simulink model "SpaceFlexibleRobotLoadAug"  (R2025b)
settings: Solver=VariableStepAuto  StartTime=0.0  StopTime=10.0  RelTol=1e-3
undefined symbols (not defined in the file): DAP0, Ignew, InvDyn, InvDynAug, Jr, ra_norm, sig4, uls, ureal, uss, uw, XI
libraries: RCTblocks x210, SDTlibV2 x5
(part 1 of 4)
settings Model: Creator=T.FORMOSA  LastModifiedBy=andre
settings SolverCC: AlgebraicLoopSolver=TrustRegion
settings DebuggingCC: AlgebraicLoopMsg=none  UnconnectedInputMsg=warning  UnconnectedOutputMsg=warning  UnconnectedLineMsg=warning  ArithmeticOperatorsInVariantConditions=warning
settings ModelReferenceCC: EnableRefExpFcnMdlSchedulingChecks=on
settings SFSimCC: CustomCodeUndefinedFunction=UseInterfaceOnly
settings RTWCC: GPUComputeCapability=3.5  DLArmComputeVersion=19.05

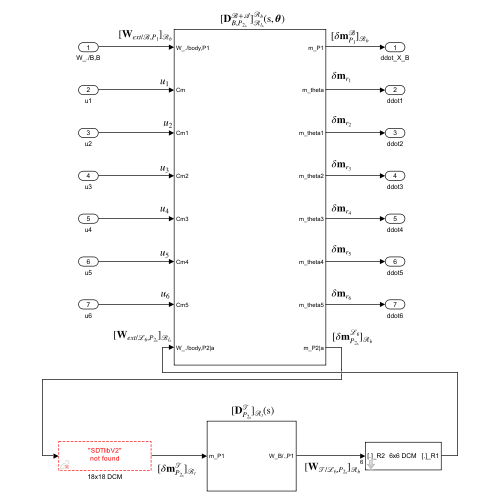
[thumbnail: Simulink's stored preview of the top-level diagram]
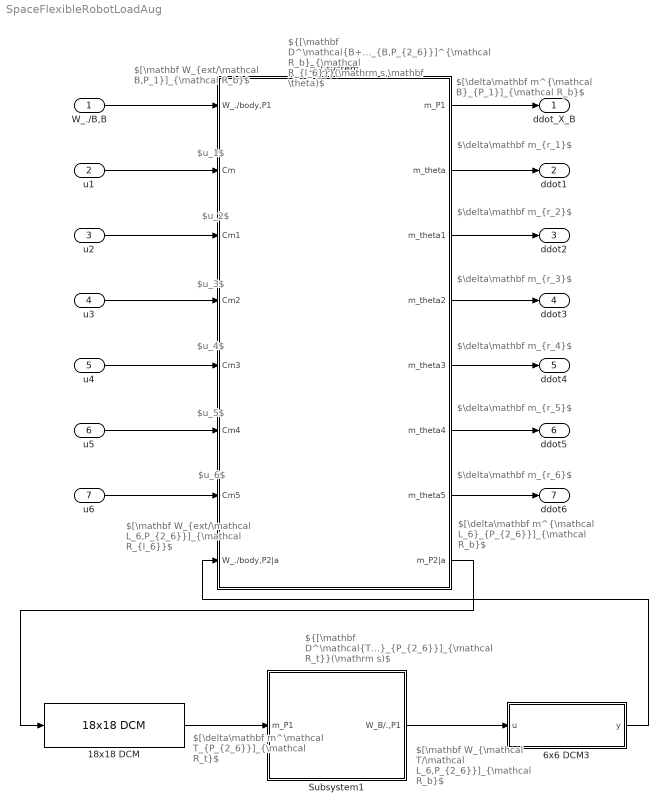
== system SpaceFlexibleRobotLoadAug ==
  note: $[\mathbf W_{ext/\mathcal B,P_1}]_{\mathcal R_b}$
  note: $[\delta\mathbf m^{\mathcal B}_{P_1}]_{\mathcal R_b}$
  note: $u_1$
  note: $\delta\mathbf m_{r_1}$
  note: $u_2$
  note: $u_3$
  note: $u_4$
  note: $u_5$
  note: $u_6$
  note: $[\mathbf W_{ext/\mathcal L_6,P_{2_6}}]_{\mathcal R_{l_6}}$
  note: $\delta\mathbf m_{r_2}$
  note: $\delta\mathbf m_{r_3}$
  note: $\delta\mathbf m_{r_4}$
  note: $\delta\mathbf m_{r_5}$
  note: $\delta\mathbf m_{r_6}$
  note: $[\delta\mathbf m^{\mathcal L_6}_{P_{2_6}}]_{\mathcal R_b}$
  note: ${[\mathbf D^\mathcal{B+A}_{B,P_{2_6}}]^{\mathcal R_b}_{\mathcal R_{l_6}}}(\mathrm s,\mathbf \theta)$
  note: $[\mathbf W_{\mathcal T/\mathcal L_6,P_{2_6}}]_{\mathcal R_b}$
  note: $[\delta\mathbf m^\mathcal T_{P_{2_6}}]_{\mathcal R_t}$
  note: ${[\mathbf D^\mathcal{T}_{P_{2_6}}]_{\mathcal R_t}}(\mathrm s)$
  W_./B,B : Inport
  u1 : Inport  Port=2
  u2 : Inport  Port=3
  u3 : Inport  Port=4
  u4 : Inport  Port=5
  u5 : Inport  Port=6
  u6 : Inport  Port=7
  18x18 DCM : SDTlibV2/3//6//18 DCM/18x18 DCM  rot=[0 0 1;-1 0 0;0 -1 0]  transp=on
      settings: SourceProductName=SDTlib
  6x6 DCM3 : Subsystem  mask(6x6 Direction cosine matrix (DCM)){rot=[0 0 1;-1 0 0;0 -1 0], transp=off}
      mask prompts: rot "3x3 DCM"; transp "Matrix transposed"
      mask help:
      | For 6 d.o.f. body motion (3 translations and 3 rotations), this block Implement the 6x6 rotation matrix (or its transposed) for a given 3x3 DCM.
      |
      | Considering 2 frames R1 and  R2, the DCM between R1 and R2 is defined as the 3x3 matrix where each column is the component vector of each R2 orthogonal unit vector expressed in R1. Thus
      |
      |    [v]_R1 = DCM  * [v]_R2.
      mask init:
      | if transp,
      |     rot=rot';
      | end
      mask Help: web('Doc6dcm.html','-browser')
      mask Display:
      | disp('6x6 DCM')
      | if transp
      |     port_label('input', 1, '[.]_R1')
      |     port_label('output', 1, '[.]_R2')
      | else
      |     port_label('input', 1, '[.]_R2')
      |     port_label('output', 1, '[.]_R1')
      | end
  Subsystem : Subsystem
  Subsystem1 : Subsystem
  ddot_X_B : Outport  VectorParamsAs1DForOutWhenUnconnected=off
  ddot1 : Outport  Port=2  VectorParamsAs1DForOutWhenUnconnected=off
  ddot2 : Outport  Port=3  VectorParamsAs1DForOutWhenUnconnected=off
  ddot3 : Outport  Port=4  VectorParamsAs1DForOutWhenUnconnected=off
  ddot4 : Outport  Port=5  VectorParamsAs1DForOutWhenUnconnected=off
  ddot5 : Outport  Port=6  VectorParamsAs1DForOutWhenUnconnected=off
  ddot6 : Outport  Port=7  VectorParamsAs1DForOutWhenUnconnected=off
  wires:
  W_./B,B/1 -> Subsystem/1(W_./body,P1)
  u1/1 -> Subsystem/2(Cm)
  u2/1 -> Subsystem/3(Cm1)
  u3/1 -> Subsystem/4(Cm2)
  u4/1 -> Subsystem/5(Cm3)
  u5/1 -> Subsystem/6(Cm4)
  u6/1 -> Subsystem/7(Cm5)
  6x6 DCM3/1(y) -> Subsystem/8(W_./body,P2|a)
  Subsystem/1(m_P1) -> ddot_X_B/1
  Subsystem/2(m_theta) -> ddot1/1
  Subsystem/3(m_theta1) -> ddot2/1
  Subsystem/4(m_theta2) -> ddot3/1
  Subsystem/5(m_theta3) -> ddot4/1
  Subsystem/6(m_theta4) -> ddot5/1
  Subsystem/7(m_theta5) -> ddot6/1
  Subsystem/8(m_P2|a) -> 18x18 DCM/1
  Subsystem1/1(W_B/.,P1) -> 6x6 DCM3/1(u)
  18x18 DCM/1 -> Subsystem1/1(m_P1)

== system SpaceFlexibleRobotLoadAug/6x6 DCM3 ==
  u : Inport  PortDimensions=6
  Demux : Demux  Outputs=[3 3]
  Mux : Mux  Inputs=[3 3]
  rotation : Gain  Gain=rot  Multiplication=Matrix(K*u) (u vector)
  translation : Gain  Gain=rot  Multiplication=Matrix(K*u) (u vector)
  y : Outport  VectorParamsAs1DForOutWhenUnconnected=off
  wires:
  rotation/1 -> Mux/2
  translation/1 -> Mux/1
  Demux/1 -> translation/1
  u/1 -> Demux/1
  Mux/1 -> y/1
  Demux/2 -> rotation/1

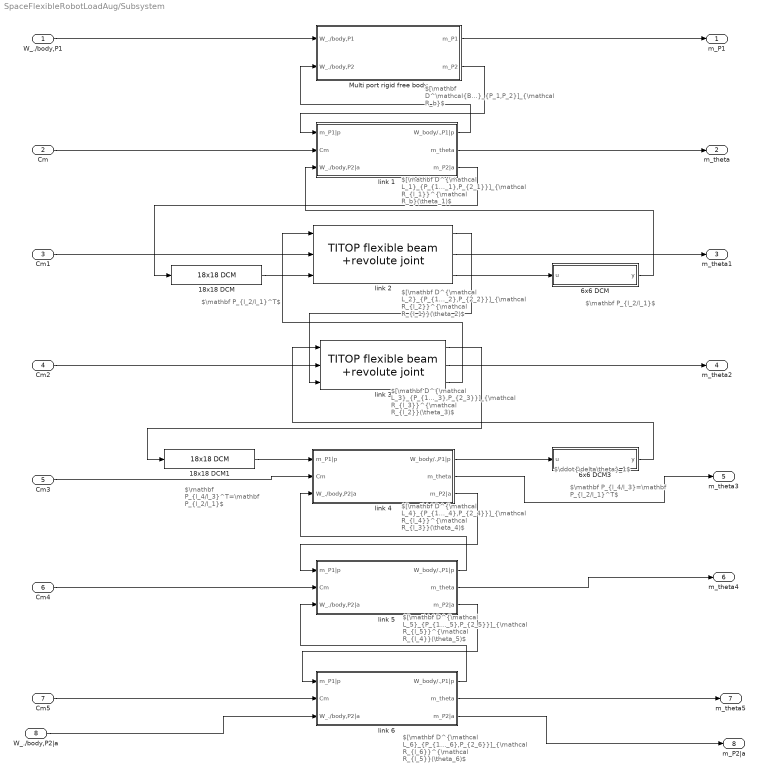
== system SpaceFlexibleRobotLoadAug/Subsystem ==
  note: $[\mathbf D^{\mathcal L_1}_{P_{1_1},P_{2_1}}]_{\mathcal R_{l_1}}^{\mathcal R_b}(\theta_1)$
  note: $[\mathbf D^\mathcal{B}_{P_1,P_2}]_{\mathcal R_b}$
  note: $\ddot{\delta\theta}_1$
  note: $[\mathbf D^{\mathcal L_2}_{P_{1_2},P_{2_2}}]_{\mathcal R_{l_2}}^{\mathcal R_{l_1}}(\theta_2)$
  note: $[\mathbf D^{\mathcal L_3}_{P_{1_3},P_{2_3}}]_{\mathcal R_{l_3}}^{\mathcal R_{l_2}}(\theta_3)$
  note: $[\mathbf D^{\mathcal L_4}_{P_{1_4},P_{2_4}}]_{\mathcal R_{l_4}}^{\mathcal R_{l_3}}(\theta_4)$
  note: $[\mathbf D^{\mathcal L_5}_{P_{1_5},P_{2_5}}]_{\mathcal R_{l_5}}^{\mathcal R_{l_4}}(\theta_5)$
  note: $[\mathbf D^{\mathcal L_6}_{P_{1_6},P_{2_6}}]_{\mathcal R_{l_6}}^{\mathcal R_{l_5}}(\theta_6)$
  note: $\mathbf P_{l_2/l_1}$
  note: $\mathbf P_{l_2/l_1}^T$
  note: $\mathbf P_{l_4/l_3}=\mathbf P_{l_2/l_1}^T$
  note: $\mathbf P_{l_4/l_3}^T=\mathbf P_{l_2/l_1}$
  W_./body,P1 : Inport
  Cm : Inport  Port=2
  Cm1 : Inport  Port=3
  Cm2 : Inport  Port=4
  Cm3 : Inport  Port=5
  Cm4 : Inport  Port=6
  Cm5 : Inport  Port=7
  W_./body,P2|a : Inport  Port=8
  18x18 DCM : SDTlibV2/3//6//18 DCM/18x18 DCM  rot=[0 1 0;-1 0 0;0 0 1]  transp=on
      settings: SourceProductName=SDTlib
  18x18 DCM1 : SDTlibV2/3//6//18 DCM/18x18 DCM  rot=[0 1 0;-1 0 0;0 0 1]  transp=off
      settings: SourceProductName=SDTlib
  6x6 DCM : Subsystem  mask(6x6 Direction cosine matrix (DCM)){rot=[0 1 0;-1 0 0;0 0 1], transp=off}
      mask prompts: rot "3x3 DCM"; transp "Matrix transposed"
      mask help:
      | For 6 d.o.f. body motion (3 translations and 3 rotations), this block Implement the 6x6 rotation matrix (or its transposed) for a given 3x3 DCM.
      |
      | Considering 2 frames R1 and  R2, the DCM between R1 and R2 is defined as the 3x3 matrix where each column is the component vector of each R2 orthogonal unit vector expressed in R1. Thus
      |
      |    [v]_R1 = DCM  * [v]_R2.
      mask init:
      | if transp,
      |     rot=rot';
      | end
      mask Help: web('Doc6dcm.html','-browser')
      mask Display:
      | disp('6x6 DCM')
      | if transp
      |     port_label('input', 1, '[.]_R1')
      |     port_label('output', 1, '[.]_R2')
      | else
      |     port_label('input', 1, '[.]_R2')
      |     port_label('output', 1, '[.]_R1')
      | end
  6x6 DCM3 : Subsystem  mask(6x6 Direction cosine matrix (DCM)){rot=[0 1 0;-1 0 0;0 0 1], transp=on}
      mask prompts: rot "3x3 DCM"; transp "Matrix transposed"
      mask help:
      | For 6 d.o.f. body motion (3 translations and 3 rotations), this block Implement the 6x6 rotation matrix (or its transposed) for a given 3x3 DCM.
      |
      | Considering 2 frames R1 and  R2, the DCM between R1 and R2 is defined as the 3x3 matrix where each column is the component vector of each R2 orthogonal unit vector expressed in R1. Thus
      |
      |    [v]_R1 = DCM  * [v]_R2.
      mask init:
      | if transp,
      |     rot=rot';
      | end
      mask Help: web('Doc6dcm.html','-browser')
      mask Display:
      | disp('6x6 DCM')
      | if transp
      |     port_label('input', 1, '[.]_R1')
      |     port_label('output', 1, '[.]_R2')
      | else
      |     port_label('input', 1, '[.]_R2')
      |     port_label('output', 1, '[.]_R1')
      | end
  Multi port rigid free body : Subsystem  mask(Multi-port rigid body (18nx6n)){m=1000, Ig=[666.6667 0 0; 0 666.6667 0; 0 0 666.6667], OG=[0;0;0], n=2, OP1=[0;0;0], OP2=[0;0;1], OP3=[ureal('P3_y',1,'percent',10);0;0], OP4=[0;0;0], OP5=[0;0;0]}
      mask prompts: m "Mass (Kg)"; Ig "Inertia (at G, Kg m^2)"; OG "OG (3x1 vector, m)"; n "Number of ports"; OP1 "OP1 (3x1 vector, m)"; OP2 "OP2 (3x1 vector, m)"; OP3 "OP3 (3x1 vector, m)"; OP4 "OP4 (3x1 vector, m)"; OP5 "OP5 (3x1 vector,m)"
      mask help:
      | 18nx6n dynamic model of a rigid body at n given points (ports) between wrenches applied at the n points (input) and the motions vectors at these points (output).
      |
      | 0: the reference point
      | G: the center of mass
      | Pi (i=1:n): the n given connection points (n<6).
      |
      | All parameters are expressed in the body frame.
      | Each parameter can be an uncertain parameter declared with "ureal"
      mask init:
      | MultiPortRigidFreeBody
      mask Help: web('Docmultiportrigidbase.html','-browser')
      mask TypeOptions n: 1 | 2 | 3 | 4 | 5
      mask DialogControl ParameterGroupVar Prompt: Main parameters
      mask DialogControl port1 Prompt: Port #1
      mask DialogControl port2 Prompt: #2
      mask DialogControl port3 Prompt: #3
      mask DialogControl port4 Prompt: #4
      mask DialogControl port5 Prompt: #5
      mask Display:
      | disp('Multi-port\n rigid free body\n (18nx6n)')
      | for ii=1:n
      |     port_label('input', ii,['W_{./body,P',num2str(ii),'}'],'interpreter','tex')
      |     port_label('output',ii,['m_{P',num2str(ii),'}'],'interpreter','tex')
      | end
  link 1 : Subsystem  mask(Multi-port rigid body with revolute joint (18n-9)x(6n+15)){m=60, Ig=[1.6 0 0; 0 1.6 0; 0 0 0.67], OG=[0;0;0.25], n=2, OP1=[0;0;0], OP2=[0;0;0.5], OP3=[0;0;0.25], OP4=[0;12;0], OP5=[0;0;0], ra=[0;0;1], theta=ureal('theta1',0,'Range',[-pi pi])}
      mask prompts: m "Mass (kg)"; Ig "Inertia at G in Ra (kg.m^2)"; OG "OG (3x1 vector in Ra)  (m)"; n "n (number of connection points)"; OP1 "OP1 (3x1 vector in Ra) (m)"; OP2 "OP2 (3x1 vector in Ra) (m)"; OP3 "OP3 (3x1 vector in Ra) (m)"; OP4 "OP4 (3x1 vector in Ra) (m)"; OP5 "OP5 (3x1 vector in Ra) (m)"; ra "ra (joint axis) (3x1 vector)"; theta "Angular configuration (rad)"
      mask help:
      | Computes the (18n-9)x(6n+13) model :
      | - 6x18 transfer from the motion vector to the wrench applied by this body to a parent body at port P1 through a revolute joint,
      | - the 3x1 channel :
      |               * from  the  joint torque applied by the input (parent) shaft to the output (body) shaft
      |               * to the relative motion vector of the output shaft w.r.t the input shaft ([thetaddot;thetadot;theta]),
      | - (n-1) 18x6 transfers from the wrenches applied to this body to the motion vectors at ports P2,P3,..,
      |
      | Input/Output of port P1 are expressed in the parent frame Rp
      | Input/Output of ports P2,P3,... are expressed in the body frame Ra.
      |
      | O: the body reference point
      | G: the center of mass
      | Pi (i=1:n): the n given connection points or ports (n<6).
      | ra: direction of the revolute joint in the Rp (or Ra)
      | theta: angular configuration of the joint (Ra is obtained from Rp by a rotation of theta around ra).
      |
      | All parameters must be expressed in the body frame Ra.
      | Each parameter can be an uncertain parameter declared with the function ureal (except ra)
      |
      | Rk: if "theta" field is: ureal('NAME',0,'Range',[-pi pi])
      | then, ULINEARIZE will provide a model involving the block named "tan_NAME_div4";
      mask init:
      | MultiPortRigidBodyRevAug
      mask Help: web('DocMultiportRigidBodyRevolute.html','-browser')
      mask TypeOptions n: 1 | 2 | 3 | 4 | 5
      mask DialogControl ParameterGroupVar Prompt: Rigid body parameter
      mask DialogControl port1 Prompt: #1
      mask DialogControl port2 Prompt: #2
      mask DialogControl port3 Prompt: #3
      mask DialogControl port4 Prompt: #4
      mask DialogControl port5 Prompt: #5
      mask DialogControl JointParameters Prompt: Revolute joint parameters
      mask Display:
      | disp('Multi-port\n rigid body\n+ revolute joint \n(18n-9)x(6n+13)')
      | 
      | port_label('input', 1,'m_P1|p')
      | port_label('output',1,'Wbody/.,P1|p')
      | port_label('input', 2,'Cm_at_P1')
      | port_label('output',2,'m_\theta at P1','interpreter','tex')
      | 
      | if n>1
      |     for i=2:n
      |         port_label('input', i+1,['W./body,P',num2str(i),'|a'])
      |         port_label('output',i+1,['m_P',num2str(i),'|a'])
      |     end
      | end
  link 2 : SDTlibV2/Predefined subsystems/TITOP flexible beam +revolute joint  l=6.4  s=2*pi*0.01*0.1  rho=2700  E=70e9  Iz=pi*(0.105^4-0.095^4)/4  Iy=pi*(0.105^4-0.095^4)/4  ni=0.35  xi=0.001  Won=off  uw_var=10  Nflex=3  ra=[0;-1;0]  theta=ureal('theta2',0,'Range',[-pi pi])
      settings: SourceProductName=SDTlib
  link 3 : SDTlibV2/Predefined subsystems/TITOP flexible beam +revolute joint  l=7  s=2*pi*0.01*0.1  rho=2700  E=70e9  Iz=pi*(0.105^4-0.095^4)/4  Iy=pi*(0.105^4-0.095^4)/4  ni=0.35  xi=0.001  Won=off  uw_var=10  Nflex=3  ra=[0;-1;0]  theta=ureal('theta3',0,'Range',[-pi pi])
      settings: SourceProductName=SDTlib
  link 4 : Subsystem  mask(Multi-port rigid body with revolute joint (18n-9)x(6n+15)){m=40, Ig=[1.55 0 0; 0 0.45 0; 0 0 1.55], OG=[0;-0.32;0], n=2, OP1=[0;0;0], OP2=[0;-0.64;0], OP3=[0;0;0.25], OP4=[0;12;0], OP5=[0;0;0], ra=[-1;0;0], theta=ureal('theta4',0,'Range',[-pi pi])}
      mask prompts: m "Mass (kg)"; Ig "Inertia at G in Ra (kg.m^2)"; OG "OG (3x1 vector in Ra)  (m)"; n "n (number of connection points)"; OP1 "OP1 (3x1 vector in Ra) (m)"; OP2 "OP2 (3x1 vector in Ra) (m)"; OP3 "OP3 (3x1 vector in Ra) (m)"; OP4 "OP4 (3x1 vector in Ra) (m)"; OP5 "OP5 (3x1 vector in Ra) (m)"; ra "ra (joint axis) (3x1 vector)"; theta "Angular configuration (rad)"
      mask help:
      | Computes the (18n-9)x(6n+13) model :
      | - 6x18 transfer from the motion vector to the wrench applied by this body to a parent body at port P1 through a revolute joint,
      | - the 3x1 channel :
      |               * from  the  joint torque applied by the input (parent) shaft to the output (body) shaft
      |               * to the relative motion vector of the output shaft w.r.t the input shaft ([thetaddot;thetadot;theta]),
      | - (n-1) 18x6 transfers from the wrenches applied to this body to the motion vectors at ports P2,P3,..,
      |
      | Input/Output of port P1 are expressed in the parent frame Rp
      | Input/Output of ports P2,P3,... are expressed in the body frame Ra.
      |
      | O: the body reference point
      | G: the center of mass
      | Pi (i=1:n): the n given connection points or ports (n<6).
      | ra: direction of the revolute joint in the Rp (or Ra)
      | theta: angular configuration of the joint (Ra is obtained from Rp by a rotation of theta around ra).
      |
      | All parameters must be expressed in the body frame Ra.
      | Each parameter can be an uncertain parameter declared with the function ureal (except ra)
      |
      | Rk: if "theta" field is: ureal('NAME',0,'Range',[-pi pi])
      | then, ULINEARIZE will provide a model involving the block named "tan_NAME_div4";
      mask init:
      | MultiPortRigidBodyRevAug
      mask Help: web('DocMultiportRigidBodyRevolute.html','-browser')
      mask TypeOptions n: 1 | 2 | 3 | 4 | 5
      mask DialogControl ParameterGroupVar Prompt: Rigid body parameter
      mask DialogControl port1 Prompt: #1
      mask DialogControl port2 Prompt: #2
      mask DialogControl port3 Prompt: #3
      mask DialogControl port4 Prompt: #4
      mask DialogControl port5 Prompt: #5
      mask DialogControl JointParameters Prompt: Revolute joint parameters
      mask Display:
      | disp('Multi-port\n rigid body\n+ revolute joint \n(18n-9)x(6n+13)')
      | 
      | port_label('input', 1,'m_P1|p')
      | port_label('output',1,'Wbody/.,P1|p')
      | port_label('input', 2,'Cm_at_P1')
      | port_label('output',2,'m_\theta at P1','interpreter','tex')
      | 
      | if n>1
      |     for i=2:n
      |         port_label('input', i+1,['W./body,P',num2str(i),'|a'])
      |         port_label('output',i+1,['m_P',num2str(i),'|a'])
      |     end
      | end
  link 5 : Subsystem  mask(Multi-port rigid body with revolute joint (18n-9)x(6n+15)){m=30, Ig=[1.16 0 0; 0 0.34 0; 0 0 1.16], OG=[0;-0.32;0], n=2, OP1=[0;0;0], OP2=[0;-0.64;0], OP3=[0;0;0.25], OP4=[0;12;0], OP5=[0;0;0], ra=[0;0;1], theta=ureal('theta5',0,'Range',[-pi pi])}
      mask prompts: m "Mass (kg)"; Ig "Inertia at G in Ra (kg.m^2)"; OG "OG (3x1 vector in Ra)  (m)"; n "n (number of connection points)"; OP1 "OP1 (3x1 vector in Ra) (m)"; OP2 "OP2 (3x1 vector in Ra) (m)"; OP3 "OP3 (3x1 vector in Ra) (m)"; OP4 "OP4 (3x1 vector in Ra) (m)"; OP5 "OP5 (3x1 vector in Ra) (m)"; ra "ra (joint axis) (3x1 vector)"; theta "Angular configuration (rad)"
      mask help:
      | Computes the (18n-9)x(6n+13) model :
      | - 6x18 transfer from the motion vector to the wrench applied by this body to a parent body at port P1 through a revolute joint,
      | - the 3x1 channel :
      |               * from  the  joint torque applied by the input (parent) shaft to the output (body) shaft
      |               * to the relative motion vector of the output shaft w.r.t the input shaft ([thetaddot;thetadot;theta]),
      | - (n-1) 18x6 transfers from the wrenches applied to this body to the motion vectors at ports P2,P3,..,
      |
      | Input/Output of port P1 are expressed in the parent frame Rp
      | Input/Output of ports P2,P3,... are expressed in the body frame Ra.
      |
      | O: the body reference point
      | G: the center of mass
      | Pi (i=1:n): the n given connection points or ports (n<6).
      | ra: direction of the revolute joint in the Rp (or Ra)
      | theta: angular configuration of the joint (Ra is obtained from Rp by a rotation of theta around ra).
      |
      | All parameters must be expressed in the body frame Ra.
      | Each parameter can be an uncertain parameter declared with the function ureal (except ra)
      |
      | Rk: if "theta" field is: ureal('NAME',0,'Range',[-pi pi])
      | then, ULINEARIZE will provide a model involving the block named "tan_NAME_div4";
      mask init:
      | MultiPortRigidBodyRevAug
      mask Help: web('DocMultiportRigidBodyRevolute.html','-browser')
      mask TypeOptions n: 1 | 2 | 3 | 4 | 5
      mask DialogControl ParameterGroupVar Prompt: Rigid body parameter
      mask DialogControl port1 Prompt: #1
      mask DialogControl port2 Prompt: #2
      mask DialogControl port3 Prompt: #3
      mask DialogControl port4 Prompt: #4
      mask DialogControl port5 Prompt: #5
      mask DialogControl JointParameters Prompt: Revolute joint parameters
      mask Display:
      | disp('Multi-port\n rigid body\n+ revolute joint \n(18n-9)x(6n+13)')
      | 
      | port_label('input', 1,'m_P1|p')
      | port_label('output',1,'Wbody/.,P1|p')
      | port_label('input', 2,'Cm_at_P1')
      | port_label('output',2,'m_\theta at P1','interpreter','tex')
      | 
      | if n>1
      |     for i=2:n
      |         port_label('input', i+1,['W./body,P',num2str(i),'|a'])
      |         port_label('output',i+1,['m_P',num2str(i),'|a'])
      |     end
      | end
  link 6 : Subsystem  mask(Multi-port rigid body with revolute joint (18n-9)x(6n+15)){m=30, Ig=[1.16 0 0; 0 0.34 0; 0 0 1.16], OG=[0;-0.32;0], n=2, OP1=[0;0;0], OP2=[0;-0.64;0], OP3=[0;0;0.25], OP4=[0;12;0], OP5=[0;0;0], ra=[0;-1;0], theta=ureal('theta6',0,'Range',[-pi pi])}
      mask prompts: m "Mass (kg)"; Ig "Inertia at G in Ra (kg.m^2)"; OG "OG (3x1 vector in Ra)  (m)"; n "n (number of connection points)"; OP1 "OP1 (3x1 vector in Ra) (m)"; OP2 "OP2 (3x1 vector in Ra) (m)"; OP3 "OP3 (3x1 vector in Ra) (m)"; OP4 "OP4 (3x1 vector in Ra) (m)"; OP5 "OP5 (3x1 vector in Ra) (m)"; ra "ra (joint axis) (3x1 vector)"; theta "Angular configuration (rad)"
      mask help:
      | Computes the (18n-9)x(6n+13) model :
      | - 6x18 transfer from the motion vector to the wrench applied by this body to a parent body at port P1 through a revolute joint,
      | - the 3x1 channel :
      |               * from  the  joint torque applied by the input (parent) shaft to the output (body) shaft
      |               * to the relative motion vector of the output shaft w.r.t the input shaft ([thetaddot;thetadot;theta]),
      | - (n-1) 18x6 transfers from the wrenches applied to this body to the motion vectors at ports P2,P3,..,
      |
      | Input/Output of port P1 are expressed in the parent frame Rp
      | Input/Output of ports P2,P3,... are expressed in the body frame Ra.
      |
      | O: the body reference point
      | G: the center of mass
      | Pi (i=1:n): the n given connection points or ports (n<6).
      | ra: direction of the revolute joint in the Rp (or Ra)
      | theta: angular configuration of the joint (Ra is obtained from Rp by a rotation of theta around ra).
      |
      | All parameters must be expressed in the body frame Ra.
      | Each parameter can be an uncertain parameter declared with the function ureal (except ra)
      |
      | Rk: if "theta" field is: ureal('NAME',0,'Range',[-pi pi])
      | then, ULINEARIZE will provide a model involving the block named "tan_NAME_div4";
      mask init:
      | MultiPortRigidBodyRevAug
      mask Help: web('DocMultiportRigidBodyRevolute.html','-browser')
      mask TypeOptions n: 1 | 2 | 3 | 4 | 5
      mask DialogControl ParameterGroupVar Prompt: Rigid body parameter
      mask DialogControl port1 Prompt: #1
      mask DialogControl port2 Prompt: #2
      mask DialogControl port3 Prompt: #3
      mask DialogControl port4 Prompt: #4
      mask DialogControl port5 Prompt: #5
      mask DialogControl JointParameters Prompt: Revolute joint parameters
      mask Display:
      | disp('Multi-port\n rigid body\n+ revolute joint \n(18n-9)x(6n+13)')
      | 
      | port_label('input', 1,'m_P1|p')
      | port_label('output',1,'Wbody/.,P1|p')
      | port_label('input', 2,'Cm_at_P1')
      | port_label('output',2,'m_\theta at P1','interpreter','tex')
      | 
      | if n>1
      |     for i=2:n
      |         port_label('input', i+1,['W./body,P',num2str(i),'|a'])
      |         port_label('output',i+1,['m_P',num2str(i),'|a'])
      |     end
      | end
  m_P1 : Outport
  m_theta : Outport  Port=2
  m_theta1 : Outport  Port=3
  m_theta2 : Outport  Port=4
  m_theta3 : Outport  Port=5
  m_theta4 : Outport  Port=6
  m_theta5 : Outport  Port=7
  m_P2|a : Outport  Port=8
  wires:
  Cm2/1 -> link 3/2
  link 3/2 -> m_theta2/1
  Cm3/1 -> link 4/2(Cm)
  W_./body,P2|a/1 -> link 6/3(W_./body,P2|a)
  Cm1/1 -> link 2/2
  Cm/1 -> link 1/2(Cm)
  Cm4/1 -> link 5/2(Cm)
  18x18 DCM1/1 -> link 4/1(m_P1|p)
  Cm5/1 -> link 6/2(Cm)
  6x6 DCM3/1(y) -> link 3/1
  link 4/1(W_body/.,P1|p) -> 6x6 DCM3/1(u)
  link 5/2(m_theta) -> m_theta4/1
  link 5/1(W_body/.,P1|p) -> link 4/3(W_./body,P2|a)
  link 3/1 -> 18x18 DCM1/1
  Multi port rigid free body/1(m_P1) -> m_P1/1
  Multi port rigid free body/2(m_P2) -> link 1/1(m_P1|p)
  link 5/3(m_P2|a) -> link 6/1(m_P1|p)
  link 1/3(m_P2|a) -> 18x18 DCM/1
  link 4/2(m_theta) -> m_theta3/1
  link 1/1(W_body/.,P1|p) -> Multi port rigid free body/2(W_./body,P2)
  link 3/3 -> link 2/1
  link 6/2(m_theta) -> m_theta5/1
  W_./body,P1/1 -> Multi port rigid free body/1(W_./body,P1)
  link 4/3(m_P2|a) -> link 5/1(m_P1|p)
  link 1/2(m_theta) -> m_theta/1
  6x6 DCM/1(y) -> link 1/3(W_./body,P2|a)
  link 6/1(W_body/.,P1|p) -> link 5/3(W_./body,P2|a)
  link 6/3(m_P2|a) -> m_P2|a/1
  link 2/2 -> m_theta1/1
  link 2/3 -> 6x6 DCM/1(u)
  link 2/1 -> link 3/3
  18x18 DCM/1 -> link 2/3

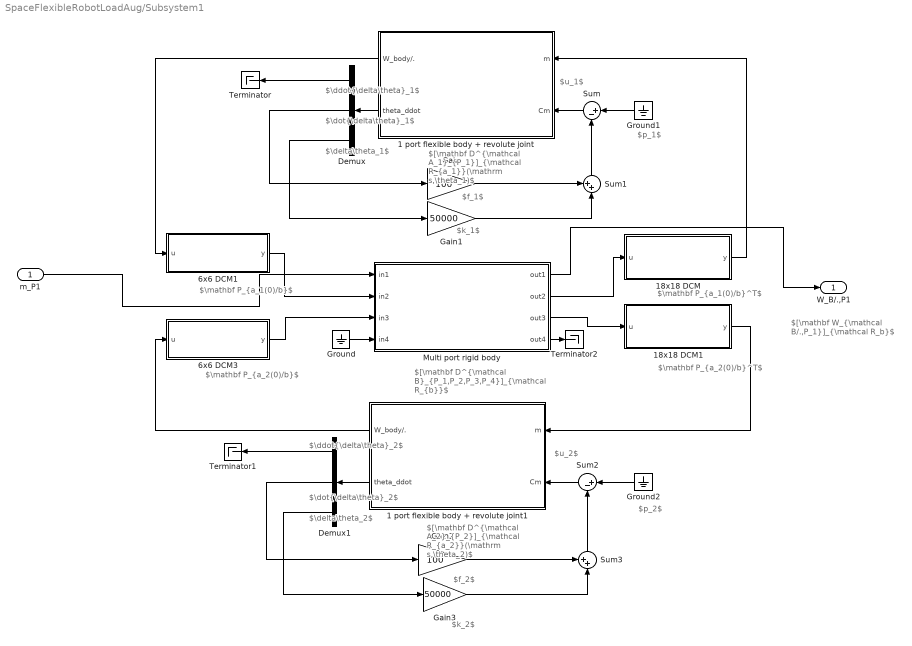
== system SpaceFlexibleRobotLoadAug/Subsystem1 ==
  note: $u_1$
  note: $\ddot{\delta\theta}_1$
  note: $\mathbf P_{a_1(0)/b}^T$
  note: $\mathbf P_{a_1(0)/b}$
  note: $\mathbf P_{a_2(0)/b}$
  note: $\mathbf P_{a_2(0)/b}^T$
  note: $\dot{\delta\theta}_1$
  note: $\dot{\delta\theta}_2$
  note: $\ddot{\delta\theta}_2$
  note: $\delta\theta_1$
  note: $\delta\theta_2$
  note: $p_1$
  note: $u_2$
  note: $p_2$
  note: $f_1$
  note: $k_1$
  note: $k_2$
  note: $f_2$
  note: $[\mathbf D^{\mathcal A_1}_{P_1}]_{\mathcal R_{a_1}}(\mathrm s,\theta_1)$
  note: $[\mathbf D^{\mathcal A_2}_{P_2}]_{\mathcal R_{a_2}}(\mathrm s,\theta_2)$
  note: $[\mathbf W_{\mathcal B/.,P_1}]_{\mathcal R_b}$
  note: $[\mathbf D^{\mathcal B}_{P_1,P_2,P_3,P_4}]_{\mathcal R_{b}}$
  m_P1 : Inport
  1 port flexible body + revolute joint : Subsystem  mask(One-port flexibe body with revolute joint (9x19)){m=43, Ig=[17 0 0;0 62 0;0 0 79], OG=[2.07;0;0], OP=[0;0;0], ra=[1;0;0], theta=ureal('Theta',0,'Range',[-pi pi]), n=3, xi=0.005, w1=5.6, L11=0, L12=0, L13=-5.12, L14=0, L15=12.5, L16=0, w2=19.3, L21=0, L22=0, L23=0, L24=-3.84, L25=0, L26=0, w3=35.4, L31=0, L32=0, L33=-2.97, L34=0, L35=2.51, L36=0, w4=2.83*2*pi, L41=0.0004, L42=-0.9132, L43=2.7900, L44=-1.8763, L45=-0.0246, L46=0.0031, w5=4.30*2*pi, L51=-0.0053, L52=5.878, L53=-1.0144, L54=3.0180, L55=-0.0124, L56=-0.0001, w6=0, L61=0, L62=0, L63=0, L64=0, L65=0, L66=0, w7=0, L71=0, L72=0, L73=0, L74=0, L75=0, L76=0, w8=0, L81=0, L82=0, L83=0, L84=0, L85=0, L86=0, w9=0, L91=0, L92=0, L93=0, L94=0, L95=0, L96=0, w10=0, L101=0, L102=0, L103=0, L104=0, L105=0, L106=0}
      mask prompts: m "Mass (Kg)"; Ig "Inertia (at G in Ra, Kgm^2)"; OG "OG (3x1 vector in Ra, m)"; OP "OP (3x1 vector in Ra, m)"; ra "ra (joint axis) (3x1 vector)"; theta "Angular configuration (rad)"; n "Number of flexible modes"; xi "Common damping ratio"; w1 "Frequency (rd/s)"; L11 "Tx (Kg^0.5)"; L12 "Ty (Kg^0.5)"; L13 "Tz (Kg^0.5)"; L14 "Rx (m.Kg^0.5)"; L15 "Ry (m.Kg^0.5)"; L16 "Rz (m.Kg^0.5)"; w2 "Frequency (rd/s)"; L21 "Tx (Kg^0.5)"; L22 "Ty (Kg^0.5)"; L23 "Tz (Kg^0.5)"; L24 "Rx (m.Kg^0.5)"; L25 "Ry (m.Kg^0.5)"; L26 "Rz (m.Kg^0.5)"; w3 "Frequency (rd/s)"; L31 "Tx (Kg^0.5)"; L32 "Ty (Kg^0.5)"; L33 "Tz (Kg^0.5)"; L34 "Rx (m.Kg^0.5)"; L35 "Ry (m.Kg^0.5)"; L36 "Rz (m.Kg^0.5)"; w4 "Frequency (rd/s)"; L41 "Tx (Kg^0.5)"; L42 "Ty (Kg^0.5)"; L43 "Tz (Kg^0.5)"; L44 "Rx (m.Kg^0.5)"; L45 "Ry (m.Kg^0.5)"; L46 "Rz (m.Kg^0.5)"; w5 "Frequency (rd/s)"; L51 "Tx (Kg^0.5)"; L52 "Ty (Kg^0.5)"; L53 "Tz (Kg^0.5)"; L54 "Rx (m.Kg^0.5)"; L55 "Ry (m.Kg^0.5)"; L56 "Rz (m.Kg^0.5)"; w6 "Frequency (rd/s)"; L61 "Tx (Kg^0.5)"; L62 "Ty (Kg^0.5)"; L63 "Tz (Kg^0.5)"; L64 "Rx (m.Kg^0.5)"; L65 "Ry (m.Kg^0.5)"; L66 "Rz (m.Kg^0.5)"; w7 "Frequency (rd/s)"; L71 "Tx (Kg^0.5)"; L72 "Ty (Kg^0.5)"; L73 "Tz (Kg^0.5)"; L74 "Rx (m.Kg^0.5)"; L75 "Ry (m.Kg^0.5)"; L76 "Rz (m.Kg^0.5)"; w8 "Frequency (rd/s)"; L81 "Tx (Kg^0.5)"; L82 "Ty (Kg^0.5)"; L83 "Tz (Kg^0.5)"; L84 "Rx (m.Kg^0.5)"; L85 "Ry (m.Kg^0.5)"; L86 "Rz (m.Kg^0.5)"; w9 "Frequency (rd/s)"; L91 "Tx (Kg^0.5)"; L92 "Ty (Kg^0.5)"; L93 "Tz (Kg^0.5)"; L94 "Rx (m.Kg^0.5)"; L95 "Ry (m.Kg^0.5)"; L96 "Rz (m.Kg^0.5)"; w10 "Frequency (rd/s)"; L101 "Tx (Kg^0.5)"; L102 "Ty (Kg^0.5)"; L103 "Tz (Kg^0.5)"; L104 "Rx (m.Kg^0.5)"; L105 "Ry (m.Kg^0.5)"; L106 "Rz (m.Kg^0.5)"
      mask help:
      | 9x19 dynamic model of a flexible body connected at point P to a parent body through a revolute joint:
      |  - 6x18 transfer from the motion vectort to the wrench applied by this body to the parent body at point P and
      |    projected in the parent body frame Rp.
      |  - the 3x1 channel  is the transfer:
      |               * from  the  joint torque applied by the input (parent) shaft to the output (body) shaft
      |               * to the relative motion vector of the output shaft w.r.t the input shaft [thetaddot;thetadot;theta].
      |
      | O: the body reference point
      | G: the center of mass
      | P: the connection point with a revolute joint
      | ra: direction of the revolute joint in the parent body frame Rp (or the flexible body frame Ra)
      |
      | All mechanical parameters are expressed in the flexible body frame Ra.
      | Each parameter can be an uncertain parameter declared with "ureal" (except ra)
      |
      | Angular configuration can be a vayring parameter: Ex:
      | ureal('NAME',0,'Range',[-pi pi])
      | Then, ULINEARIZE will provide a model involving the block named "tan_NAME_div4".
      mask init:
      | FlexBodyRev1Port
      mask Help: web('Doconeportflexrevolute.html','-browser')
      mask TypeOptions n: 0 | 1 | 2 | 3 | 4 | 5 | 6 | 7 | 8 | 9 | 10
      mask DialogControl ParameterGroupVar Prompt: Main parameters
      mask DialogControl damping Prompt: Damping ratio
      mask DialogControl mode1 Prompt: Flexible mode #1:
      mask DialogControl Control8 Prompt: Modal participation factor at P in Ra
      mask DialogControl mode2 Prompt: #2:
      mask DialogControl Control9 Prompt: Modal participation factor at P in Ra
      mask DialogControl mode3 Prompt: #3
      mask DialogControl Control10 Prompt: Modal participation factor at P in Ra
      mask DialogControl mode4 Prompt: #4
      mask DialogControl Control11 Prompt: Modal participation factor at P in Ra
      mask DialogControl mode5 Prompt: #5
      mask DialogControl Control12 Prompt: Modal participation factor at P in Ra
      mask DialogControl mode6 Prompt: #6
      mask DialogControl Control13 Prompt: Modal participation factor at P in Ra
      mask DialogControl mode7 Prompt: #7
      mask DialogControl Control14 Prompt: Modal participation factor at P in Ra
      mask DialogControl mode8 Prompt: #8
      mask DialogControl Control15 Prompt: Modal participation factor at P in Ra
      mask DialogControl mode9 Prompt: #9
      mask DialogControl Control16 Prompt: Modal participation factor at P in Ra
      mask DialogControl mode10 Prompt: #10
      mask DialogControl Control17 Prompt: Modal participation factor at P in Ra
      mask Display:
      | disp('One-port\n flexible body\n + revolute joint\n (9x19)')
      | port_label('input', 1, 'm')
      | port_label('output', 1, 'Wbody/.')
      | port_label('input', 2, 'Cm')
      | port_label('output', 2, 'm_\theta','interpreter','tex')
  1 port flexible body + revolute joint1 : Subsystem  mask(One-port flexibe body with revolute joint (9x19)){m=43, Ig=[17 0 0;0 62 0;0 0 79], OG=[2.07;0;0], OP=[0;0;0], ra=[-1;0;0], theta=ureal('Theta',0,'Range',[-pi pi]), n=3, xi=0.005, w1=5.6, L11=0, L12=0, L13=-5.12, L14=0, L15=12.5, L16=0, w2=19.3, L21=0, L22=0, L23=0, L24=-3.84, L25=0, L26=0, w3=35.4, L31=0, L32=0, L33=-2.97, L34=0, L35=2.51, L36=0, w4=2.83*2*pi, L41=0.0004, L42=-0.9132, L43=2.7900, L44=-1.8763, L45=-0.0246, L46=0.0031, w5=4.30*2*pi, L51=-0.0053, L52=5.878, L53=-1.0144, L54=3.0180, L55=-0.0124, L56=-0.0001, w6=0, L61=0, L62=0, L63=0, L64=0, L65=0, L66=0, w7=0, L71=0, L72=0, L73=0, L74=0, L75=0, L76=0, w8=0, L81=0, L82=0, L83=0, L84=0, L85=0, L86=0, w9=0, L91=0, L92=0, L93=0, L94=0, L95=0, L96=0, w10=0, L101=0, L102=0, L103=0, L104=0, L105=0, L106=0}
      mask prompts: m "Mass (Kg)"; Ig "Inertia (at G in Ra, Kgm^2)"; OG "OG (3x1 vector in Ra, m)"; OP "OP (3x1 vector in Ra, m)"; ra "ra (joint axis) (3x1 vector)"; theta "Angular configuration (rad)"; n "Number of flexible modes"; xi "Common damping ratio"; w1 "Frequency (rd/s)"; L11 "Tx (Kg^0.5)"; L12 "Ty (Kg^0.5)"; L13 "Tz (Kg^0.5)"; L14 "Rx (m.Kg^0.5)"; L15 "Ry (m.Kg^0.5)"; L16 "Rz (m.Kg^0.5)"; w2 "Frequency (rd/s)"; L21 "Tx (Kg^0.5)"; L22 "Ty (Kg^0.5)"; L23 "Tz (Kg^0.5)"; L24 "Rx (m.Kg^0.5)"; L25 "Ry (m.Kg^0.5)"; L26 "Rz (m.Kg^0.5)"; w3 "Frequency (rd/s)"; L31 "Tx (Kg^0.5)"; L32 "Ty (Kg^0.5)"; L33 "Tz (Kg^0.5)"; L34 "Rx (m.Kg^0.5)"; L35 "Ry (m.Kg^0.5)"; L36 "Rz (m.Kg^0.5)"; w4 "Frequency (rd/s)"; L41 "Tx (Kg^0.5)"; L42 "Ty (Kg^0.5)"; L43 "Tz (Kg^0.5)"; L44 "Rx (m.Kg^0.5)"; L45 "Ry (m.Kg^0.5)"; L46 "Rz (m.Kg^0.5)"; w5 "Frequency (rd/s)"; L51 "Tx (Kg^0.5)"; L52 "Ty (Kg^0.5)"; L53 "Tz (Kg^0.5)"; L54 "Rx (m.Kg^0.5)"; L55 "Ry (m.Kg^0.5)"; L56 "Rz (m.Kg^0.5)"; w6 "Frequency (rd/s)"; L61 "Tx (Kg^0.5)"; L62 "Ty (Kg^0.5)"; L63 "Tz (Kg^0.5)"; L64 "Rx (m.Kg^0.5)"; L65 "Ry (m.Kg^0.5)"; L66 "Rz (m.Kg^0.5)"; w7 "Frequency (rd/s)"; L71 "Tx (Kg^0.5)"; L72 "Ty (Kg^0.5)"; L73 "Tz (Kg^0.5)"; L74 "Rx (m.Kg^0.5)"; L75 "Ry (m.Kg^0.5)"; L76 "Rz (m.Kg^0.5)"; w8 "Frequency (rd/s)"; L81 "Tx (Kg^0.5)"; L82 "Ty (Kg^0.5)"; L83 "Tz (Kg^0.5)"; L84 "Rx (m.Kg^0.5)"; L85 "Ry (m.Kg^0.5)"; L86 "Rz (m.Kg^0.5)"; w9 "Frequency (rd/s)"; L91 "Tx (Kg^0.5)"; L92 "Ty (Kg^0.5)"; L93 "Tz (Kg^0.5)"; L94 "Rx (m.Kg^0.5)"; L95 "Ry (m.Kg^0.5)"; L96 "Rz (m.Kg^0.5)"; w10 "Frequency (rd/s)"; L101 "Tx (Kg^0.5)"; L102 "Ty (Kg^0.5)"; L103 "Tz (Kg^0.5)"; L104 "Rx (m.Kg^0.5)"; L105 "Ry (m.Kg^0.5)"; L106 "Rz (m.Kg^0.5)"
      mask help:
      | 9x19 dynamic model of a flexible body connected at point P to a parent body through a revolute joint:
      |  - 6x18 transfer from the motion vectort to the wrench applied by this body to the parent body at point P and
      |    projected in the parent body frame Rp.
      |  - the 3x1 channel  is the transfer:
      |               * from  the  joint torque applied by the input (parent) shaft to the output (body) shaft
      |               * to the relative motion vector of the output shaft w.r.t the input shaft [thetaddot;thetadot;theta].
      |
      | O: the body reference point
      | G: the center of mass
      | P: the connection point with a revolute joint
      | ra: direction of the revolute joint in the parent body frame Rp (or the flexible body frame Ra)
      |
      | All mechanical parameters are expressed in the flexible body frame Ra.
      | Each parameter can be an uncertain parameter declared with "ureal" (except ra)
      |
      | Angular configuration can be a vayring parameter: Ex:
      | ureal('NAME',0,'Range',[-pi pi])
      | Then, ULINEARIZE will provide a model involving the block named "tan_NAME_div4".
      mask init:
      | FlexBodyRev1Port
      mask Help: web('Doconeportflexrevolute.html','-browser')
      mask TypeOptions n: 0 | 1 | 2 | 3 | 4 | 5 | 6 | 7 | 8 | 9 | 10
      mask DialogControl ParameterGroupVar Prompt: Main parameters
      mask DialogControl damping Prompt: Damping ratio
      mask DialogControl mode1 Prompt: Flexible mode #1:
      mask DialogControl Control8 Prompt: Modal participation factor at P in Ra
      mask DialogControl mode2 Prompt: #2:
      mask DialogControl Control9 Prompt: Modal participation factor at P in Ra
      mask DialogControl mode3 Prompt: #3
      mask DialogControl Control10 Prompt: Modal participation factor at P in Ra
      mask DialogControl mode4 Prompt: #4
      mask DialogControl Control11 Prompt: Modal participation factor at P in Ra
      mask DialogControl mode5 Prompt: #5
      mask DialogControl Control12 Prompt: Modal participation factor at P in Ra
      mask DialogControl mode6 Prompt: #6
      mask DialogControl Control13 Prompt: Modal participation factor at P in Ra
      mask DialogControl mode7 Prompt: #7
      mask DialogControl Control14 Prompt: Modal participation factor at P in Ra
      mask DialogControl mode8 Prompt: #8
      mask DialogControl Control15 Prompt: Modal participation factor at P in Ra
      mask DialogControl mode9 Prompt: #9
      mask DialogControl Control16 Prompt: Modal participation factor at P in Ra
      mask DialogControl mode10 Prompt: #10
      mask DialogControl Control17 Prompt: Modal participation factor at P in Ra
      mask Display:
      | disp('One-port\n flexible body\n + revolute joint\n (9x19)')
      | port_label('input', 1, 'm')
      | port_label('output', 1, 'Wbody/.')
      | port_label('input', 2, 'Cm')
      | port_label('output', 2, 'm_\theta','interpreter','tex')
  18x18 DCM : Subsystem  mask(18x18 Direction cosine matrix (DCM)){rot=[0 -1 0;0 0 -1;1 0 0], transp=on}
      mask prompts: rot "3x3 DCM"; transp "Matrix transposed"
      mask help:
      | For 6 d.o.f. body motion vector (3 translations and 3 rotations, accelerations, velocities and positions), this block Implement the 18x18 rotation matrix (or its transposed) for a given 3x3 DCM.
      |
      | Considering 2 frames R1 and  R2, the DCM between R1 and R2 is defined as the 3x3 matrix where each column is the component vector of each R2 orthogonal unit vector expressed in R1. Thus
      |
      |    [v]_R1 = DCM  * [v]_R2.
      mask init:
      | if transp,
      |     rot=rot';
      | end
      mask Help: web('Doc18dcm.html','-browser')
      mask Display:
      | disp('18x18 DCM')
      | if transp
      |     port_label('input', 1, '[.]_R1')
      |     port_label('output', 1, '[.]_R2')
      | else
      |     port_label('input', 1, '[.]_R2')
      |     port_label('output', 1, '[.]_R1')
      | end
  18x18 DCM1 : Subsystem  mask(18x18 Direction cosine matrix (DCM)){rot=[0 1 0;0 0 -1;-1 0 0], transp=on}
      mask prompts: rot "3x3 DCM"; transp "Matrix transposed"
      mask help:
      | For 6 d.o.f. body motion vector (3 translations and 3 rotations, accelerations, velocities and positions), this block Implement the 18x18 rotation matrix (or its transposed) for a given 3x3 DCM.
      |
      | Considering 2 frames R1 and  R2, the DCM between R1 and R2 is defined as the 3x3 matrix where each column is the component vector of each R2 orthogonal unit vector expressed in R1. Thus
      |
      |    [v]_R1 = DCM  * [v]_R2.
      mask init:
      | if transp,
      |     rot=rot';
      | end
      mask Help: web('Doc18dcm.html','-browser')
      mask Display:
      | disp('18x18 DCM')
      | if transp
      |     port_label('input', 1, '[.]_R1')
      |     port_label('output', 1, '[.]_R2')
      | else
      |     port_label('input', 1, '[.]_R2')
      |     port_label('output', 1, '[.]_R1')
      | end
  6x6 DCM1 : Subsystem  mask(6x6 Direction cosine matrix (DCM)){rot=[0 -1 0;0 0 -1;1 0 0], transp=off}
      mask prompts: rot "3x3 DCM"; transp "Matrix transposed"
      mask help:
      | For 6 d.o.f. body motion (3 translations and 3 rotations), this block Implement the 6x6 rotation matrix (or its transposed) for a given 3x3 DCM.
      |
      | Considering 2 frames R1 and  R2, the DCM between R1 and R2 is defined as the 3x3 matrix where each column is the component vector of each R2 orthogonal unit vector expressed in R1. Thus
      |
      |    [v]_R1 = DCM  * [v]_R2.
      mask init:
      | if transp,
      |     rot=rot';
      | end
      mask Help: web('Doc6dcm.html','-browser')
      mask Display:
      | disp('6x6 DCM')
      | if transp
      |     port_label('input', 1, '[.]_R1')
      |     port_label('output', 1, '[.]_R2')
      | else
      |     port_label('input', 1, '[.]_R2')
      |     port_label('output', 1, '[.]_R1')
      | end
  6x6 DCM3 : Subsystem  mask(6x6 Direction cosine matrix (DCM)){rot=[0 1 0;0 0 -1;-1 0 0], transp=off}
      mask prompts: rot "3x3 DCM"; transp "Matrix transposed"
      mask help:
      | For 6 d.o.f. body motion (3 translations and 3 rotations), this block Implement the 6x6 rotation matrix (or its transposed) for a given 3x3 DCM.
      |
      | Considering 2 frames R1 and  R2, the DCM between R1 and R2 is defined as the 3x3 matrix where each column is the component vector of each R2 orthogonal unit vector expressed in R1. Thus
      |
      |    [v]_R1 = DCM  * [v]_R2.
      mask init:
      | if transp,
      |     rot=rot';
      | end
      mask Help: web('Doc6dcm.html','-browser')
      mask Display:
      | disp('6x6 DCM')
      | if transp
      |     port_label('input', 1, '[.]_R1')
      |     port_label('output', 1, '[.]_R2')
      | else
      |     port_label('input', 1, '[.]_R2')
      |     port_label('output', 1, '[.]_R1')
      | end
  Demux : Demux  Outputs=3
  Demux1 : Demux  Outputs=3
  Gain : Gain  Gain=100
  Gain1 : Gain  Gain=50000
  Gain2 : Gain  Gain=100
  Gain3 : Gain  Gain=50000
  Ground : Ground
  Ground1 : Ground
  Ground2 : Ground
  Multi port rigid body : Subsystem  mask(Multi-port rigid body (18(n-1)+6]x[6(n-1)+18])){m=1000, Ig=[75 1 2;1 40 -1;2 -1 80], OG=[0.35;1.5;0.5], n=4, numinv=1, OP1=[0.4;1.4;1], OP2=[0.4;1.4;1], OP3=[0.4;1.4;0], OP4=[0.35;1.5;0.5], OP5=[0;0;0]}
      mask prompts: m "Mass (Kg)"; Ig "Inertia (at G, Kg m^2)"; OG "OG (3x1 vector, m)"; n "Number of ports"; numinv "The single parent port"; OP1 "OP1 (3x1 vector, m)"; OP2 "OP2 (3x1 vector, m)"; OP3 "OP3 (3x1 vector, m)"; OP4 "OP4 (3x1 vector, m)"; OP5 "OP5 (3x1 vector,m)"
      mask help:
      | [18(n-1)+6]x[6(n-1)+18] dynamic model of a rigid body at n given points (ports) between:
      | * the wrenches applied at the n-1 child ports and  the motion vector at a single parent port (inputs).
      | * the motions vectors at the  n-1 child ports and the wrench applied by the rigid body at the parent port (output)
      |
      | 0: the reference point
      | G: the center of mass
      | Pi (i=1:n): the n given connection points (n<6).
      |
      | All parameters are expressed in the body frame.
      | Each parameter can be an uncertain parameter declared with "ureal"
      |
      | The 6x18 channel associated to the single parent port can be any of the ports.
      mask init:
      | MultiPortRigidBodyAug
      mask Help: web('Docmultiportrigidbody.html','-browser')
      mask TypeOptions n: 1 | 2 | 3 | 4 | 5
      mask TypeOptions numinv: 1 | 2 | 3 | 4 | 5
      mask DialogControl ParameterGroupVar Prompt: Main parameters
      mask DialogControl port1 Prompt: Port #1
      mask DialogControl port2 Prompt: #2
      mask DialogControl port3 Prompt: #3
      mask DialogControl port4 Prompt: #4
      mask DialogControl port5 Prompt: #5
      mask Display:
      | disp('Multi-port\n rigid body\n [18(n-1)+6]x[6(n-1)+18]')
      | if n==1,
      |     if numinv==1,
      |         port_label('input', 1,'m_P')
      |         port_label('output',1,'Wbody/.,P')
      |     else
      |         port_label('input', 1,'W./body,P')
      |         port_label('output',1,'m_P')
      |     end
      | else
      |     for ii=1:n
      |         if numinv==ii,
      |             port_label('output',ii,['Wbody/.,P',num2str(ii)])
      |             port_label('input', ii,['m_P',num2str(ii)])
      |         else
      |             port_label('input', ii,['W./body,P',num2str(ii)])
      |             port_label('output',ii,['m_P',num2str(ii)])
      |         end
      |     end
      | end
  Sum : Sum  Inputs=|+-
  Sum1 : Sum  Inputs=++|
  Sum2 : Sum  Inputs=|+-
  Sum3 : Sum  Inputs=++|
  Terminator : Terminator
  Terminator1 : Terminator
  Terminator2 : Terminator
  W_B/.,P1 : Outport
  wires:
  m_P1/1 -> Multi port rigid body/1(in1)
  Gain2/1 -> Sum3/1
  Sum/1 -> 1 port flexible body + revolute joint/2(Cm)
  1 port flexible body + revolute joint1/1(W_body/.) -> 6x6 DCM3/1(u)
  Demux1/1 -> Terminator1/1
  6x6 DCM1/1(y) -> Multi port rigid body/2(in2)
  Demux/3 -> Gain1/1
  1 port flexible body + revolute joint1/2(theta_ddot) -> Demux1/1
  Ground/1 -> Multi port rigid body/4(in4)
  Ground2/1 -> Sum2/1
  Gain3/1 -> Sum3/2
  Sum1/1 -> Sum/2
  Demux1/3 -> Gain3/1
  18x18 DCM/1(y) -> 1 port flexible body + revolute joint/1(m)
  Demux/1 -> Terminator/1
  Multi port rigid body/4(out4) -> Terminator2/1
  Demux1/2 -> Gain2/1
  Sum2/1 -> 1 port flexible body + revolute joint1/2(Cm)
  6x6 DCM3/1(y) -> Multi port rigid body/3(in3)
  Multi port rigid body/1(out1) -> W_B/.,P1/1
  Multi port rigid body/2(out2) -> 18x18 DCM/1(u)
  Gain/1 -> Sum1/1
  Gain1/1 -> Sum1/2
  1 port flexible body + revolute joint/1(W_body/.) -> 6x6 DCM1/1(u)
  Ground1/1 -> Sum/1
  Multi port rigid body/3(out3) -> 18x18 DCM1/1(u)
  1 port flexible body + revolute joint/2(theta_ddot) -> Demux/1
  18x18 DCM1/1(y) -> 1 port flexible body + revolute joint1/1(m)
  Demux/2 -> Gain/1
  Sum3/1 -> Sum2/2

== system SpaceFlexibleRobotLoadAug/Subsystem/6x6 DCM ==
  u : Inport  PortDimensions=6
  Demux : Demux  Outputs=[3 3]
  Mux : Mux  Inputs=[3 3]
  rotation : Gain  Gain=rot  Multiplication=Matrix(K*u) (u vector)
  translation : Gain  Gain=rot  Multiplication=Matrix(K*u) (u vector)
  y : Outport  VectorParamsAs1DForOutWhenUnconnected=off
  wires:
  rotation/1 -> Mux/2
  translation/1 -> Mux/1
  Demux/1 -> translation/1
  u/1 -> Demux/1
  Mux/1 -> y/1
  Demux/2 -> rotation/1

== system SpaceFlexibleRobotLoadAug/Subsystem/6x6 DCM3 ==
  u : Inport  PortDimensions=6
  Demux : Demux  Outputs=[3 3]
  Mux : Mux  Inputs=[3 3]
  rotation : Gain  Gain=rot  Multiplication=Matrix(K*u) (u vector)
  translation : Gain  Gain=rot  Multiplication=Matrix(K*u) (u vector)
  y : Outport  VectorParamsAs1DForOutWhenUnconnected=off
  wires:
  rotation/1 -> Mux/2
  translation/1 -> Mux/1
  Demux/1 -> translation/1
  u/1 -> Demux/1
  Mux/1 -> y/1
  Demux/2 -> rotation/1

== system SpaceFlexibleRobotLoadAug/Subsystem/Multi port rigid free body ==
  W_./body,P1 : Inport  PortDimensions=6
  W_./body,P2 : Inport  Port=2  PortDimensions=6
  Demux : Demux  Outputs=[18 18]
  Gain : RCTblocks/Uncertain State Space  Tag=USS  USystem=uss(InvDyn)  UValue=[]  X0=[]  uX0=[]
  Mux : Mux  Inputs=[6 6]
  m_P1 : Outport
  m_P2 : Outport  Port=2
  wires:
  Mux/1 -> Gain/1
  Gain/1 -> Demux/1
  W_./body,P1/1 -> Mux/1
  Demux/1 -> m_P1/1
  W_./body,P2/1 -> Mux/2
  Demux/2 -> m_P2/1

== system SpaceFlexibleRobotLoadAug/Subsystem/link 1 ==
  m_P1|p : Inport
  Cm : Inport  Port=2
  W_./body,P2|a : Inport  Port=3
  Multi port rigid body : Subsystem  mask(Multi-port rigid body (6nx6n)){m=m, Ig=Ignew, OG=OG, n=2, numinv=1, OP1=[0;0;0], OP2=[0;0;0.5], OP3=[0;0;0.25], OP4=[0;12;0], OP5=[0;0;0]}
      mask prompts: m "Mass (Kg)"; Ig "Inertia (at G, Kg m^2)"; OG "OG (3x1 vector, m)"; n "Number of ports"; numinv "Port to be inverted"; OP1 "OP1 (3x1 vector, m)"; OP2 "OP2 (3x1 vector, m)"; OP3 "OP3 (3x1 vector, m)"; OP4 "OP4 (3x1 vector, m)"; OP5 "OP5 (3x1 vector,m)"
      mask help:
      | 6nx6n dynamic model of a rigid body at n given points (ports) between wrenches applied at the n points (input) and acceleration twists at these points (output).
      |
      | 0: the reference point
      | G: the center of mass
      | Pi (i=1:n): the n given connection points (n<6).
      |
      | All parameters are expressed in the body frame.
      | Each parameter can be an uncertain parameter declared with "ureal"
      |
      | The 6x6 channel associated to one port can be inverted: then the input of this channel is the acceleration twist imposed at this point and the output is the wrench applied by this body.
      mask init:
      | MultiPortRigidBodyAug
      mask Help: web('Docmultiportrigidbody.html','-browser')
      mask TypeOptions n: 1 | 2 | 3 | 4 | 5
      mask TypeOptions numinv: 1 | 2 | 3 | 4 | 5
      mask DialogControl ParameterGroupVar Prompt: Main parameters
      mask DialogControl port1 Prompt: Port #1
      mask DialogControl port2 Prompt: #2
      mask DialogControl port3 Prompt: #3
      mask DialogControl port4 Prompt: #4
      mask DialogControl port5 Prompt: #5
      mask Display:
      | disp('Multi-port\n rigid body\n [18(n-1)+6]x[6(n-1)+18])')
      | if n==1,
      |     if numinv==1,
      |         port_label('input', 1,'m_P')
      |         port_label('output',1,'W_body/.,P')
      |     else
      |         port_label('input', 1,'W_./body,P')
      |         port_label('output',1,'m_P')
      |     end
      | else
      |     for ii=1:n
      |         if numinv==ii,
      |             port_label('output',ii,['W_body/.,P',num2str(ii)])
      |             port_label('input', ii,['m_P',num2str(ii)])
      |         else
      |             port_label('input', ii,['W_./body,P',num2str(ii)])
      |             port_label('output',ii,['m_P',num2str(ii)])
      |         end
      |     end
      | end
  Revolute joint + configuration : Subsystem  mask(Revolute joint){ra=ra_norm, Jr=Jr, theta=theta}
      mask prompts: ra "Direction of the joint in the local frame (3x1 vector)"; Jr "Rotor inertia (kg.m^2)"; theta "Angular configuration (rad)"
      mask help:
      | This block implement the TITOP model of of a revolute joint.
      | The last channel is the transfer between the torque applied inside the joint by the input shaft to the output shaft and the relative angular acceleration of the output shaft w.r.t the input shaft.
      |
      | Angular configuration can be a vayring parameter: Ex:
      | ureal('NAME',0,'Range',[-pi pi])
      |
      | Then, ULINEARIZE will provide a model involving the block named "tan_NAME_div4";
      mask init:
      | pass=ra2DCMi(ra);
      | ran=[ra(1);ra(2);ra(3)]/norm(ra);
      mask Help: web('DocRevoluteJoint_configuration.html','-browser')
      mask Display:
      | disp('Revolute joint\nTITOP model\n+ angle configuration')
      | port_label('input', 1, 'W_./r_out|a')
      | port_label('output', 1, 'm_out|a')
      | port_label('input', 2, 'm_in|p')
      | port_label('output', 2, 'W_r_in/.|p')
      | port_label('input', 3, 'Cm')
      | port_label('output', 3, 'm_\theta','interpreter','tex')
  W_body/.,P1|p : Outport  VectorParamsAs1DForOutWhenUnconnected=off
  m_theta : Outport  Port=2  VectorParamsAs1DForOutWhenUnconnected=off
  m_P2|a : Outport  Port=3
  wires:
  Revolute joint + configuration/1(m_out|a) -> Multi port rigid body/1(in1)
  Multi port rigid body/1(out1) -> Revolute joint + configuration/1(W_./r_out|a)
  m_P1|p/1 -> Revolute joint + configuration/2(m_in|p)
  Cm/1 -> Revolute joint + configuration/3(Cm)
  Revolute joint + configuration/2(W_r_in/.|p) -> W_body/.,P1|p/1
  Revolute joint + configuration/3(m_theta) -> m_theta/1
  W_./body,P2|a/1 -> Multi port rigid body/2(in2)
  Multi port rigid body/2(out2) -> m_P2|a/1
